simulink model "spot410_savedOnboard"  (R2024b)
settings: Solver=ode4  StartTime=0.0  StopTime=tsim  FixedStep=baseRate  RelTol=1e-6  AbsTol=1e-6
values from neighbouring files (symbols this model uses):
  baseRate = paramEst(phase,coord).k1    [SpotEstimator.m]
  Gamma1_el = 0.12    [initSpotDefaultParam.m]
  Gamma1_sh = 0.005    [initSpotDefaultParam.m]
  Gamma1_wr = 0.025    [initSpotDefaultParam.m]
  Gamma2_el = 5    [initSpotDefaultParam.m]
  Gamma2_sh = 5    [initSpotDefaultParam.m]
  Gamma2_wr = 5    [initSpotDefaultParam.m]
  Gamma3_el = 10    [initSpotDefaultParam.m]
  Gamma3_sh = 40    [initSpotDefaultParam.m]
  Gamma3_wr = 40    [initSpotDefaultParam.m]
  Gamma4_el = 0.039    [initSpotDefaultParam.m]
  Gamma4_sh = 0.015    [initSpotDefaultParam.m]
  Gamma4_wr = 0.029    [initSpotDefaultParam.m]
  Gamma5_el = 800    [initSpotDefaultParam.m]
  Gamma5_sh = 800    [initSpotDefaultParam.m]
  Gamma5_wr = 800    [initSpotDefaultParam.m]
  Gamma6_el = 0.000001    (= 1e-06)    [initSpotDefaultParam.m]
  Gamma6_sh = 0.005    [initSpotDefaultParam.m]
  Gamma6_wr = 0.02    [initSpotDefaultParam.m]
  Kd_elarm = 0.8    [initSpotDefaultParam.m]
  Kd_sharm = 1.0    (= 1)    [initSpotDefaultParam.m]
  Kd_wrarm = 0.6    [initSpotDefaultParam.m]
  Kp_elarm = 1.2    [initSpotDefaultParam.m]
  Kp_sharm = 1.5    [initSpotDefaultParam.m]
  Kp_wrarm = 1.0    (= 1)    [initSpotDefaultParam.m]
  PWMFreq = 5    [initSpotDefaultParam.m]
  Tz_lim_elarm = .1    (= 0.1)    [initSpotDefaultParam.m]
  Tz_lim_sharm = .1    (= 0.1)    [initSpotDefaultParam.m]
  Tz_lim_wrarm = .1    (= 0.1)    [initSpotDefaultParam.m]
undefined symbols (not defined in the file or in its folder): a1, a2, a3, b0, b1, b2, b3, dataRate, DiscIntNeverNeededParam, drop_states_ARM, drop_states_BLACK, drop_states_BLUE, drop_states_RED, F_black_X_nominal, F_black_Y_nominal, F_blue_X_nominal, F_blue_Y_nominal, F_red_X_nominal, F_red_Y_nominal, F_thrusters_BLACK, F_thrusters_BLUE, F_thrusters_RED, home_states_BLACK, home_states_BLUE, home_states_RED, IBLACK, IBLUE, IDIST, IEE, init_states_BLACK, init_states_BLUE, init_states_RED, IPROX, IRED, K_BLACK, K_BLUE, K_RED, Kd_tb, Kd_tblue, Kd_tr, Kd_xb, Kd_xblue, Kd_xr, Kd_yb, Kd_yblue, Kd_yr, Kp_tb, Kp_tblue, Kp_tr, Kp_xb, Kp_xblue, Kp_xr, Kp_yb, Kp_yblue, Kp_yr, mBLACK, mBLUE, mDIST, mEE, mPROX ... (+21)
libraries: simulink x30, nvidiaSharedBlocks x19, MainLibrary x5, dspinverses x3, nvidiaIMUSensorslib x1
(part 8 of 8)

== matlab function spot410_savedOnboard/Thruster Control Code/Change BLUE Behavior/Calculate Duty Cycle/MATLAB Function5 ==
  data: H_final output; u_desired input; duty_cycles output; x0 input; thruster_dist2CG_BLUE parameter; F_blue_X_nominal parameter; F_blue_Y_nominal parameter; max_iters parameter; tol parameter
function [H_final,duty_cycles] = optimize_duty_cycle_with_decay(u_desired, x0, thruster_dist2CG_BLUE, F_blue_X_nominal, F_blue_Y_nominal, max_iters, tol)
    % Optimizes thruster duty cycles with decay factor updates
    %
    % Inputs:
    %   u_desired - Desired force and torque vector [Fx; Fy; M] (3x1)
    %   x0 - Initial guess for duty cycles (vector, 8x1)
    %   max_iters - Maximum number of iterations for convergence
    %   tol - Convergence tolerance for duty cycles
    %   thruster_dist2CG_BLUE - Distances of thrusters from CG (vector, mm)
    %   F_red_X_nominal - Nominal X thruster force (scalar, N)
    %   F_red_Y_nominal - Nominal Y thruster force (scalar, N)
    %
    % Outputs:
    %   duty_cycles - Optimal duty cycles for each thruster (vector, 8x1)

    % Initialization
    num_thrusters = length(x0);
    duty_cycles = x0; % Start with the initial guess
    thrust_decay_factor = 1; % Initial decay factor
    prev_duty_cycles = duty_cycles + 2 * tol; % Ensure loop starts

    % Iterative optimization process
    for iter = 1:max_iters
        % Update H matrix based on the current decay factor
        H = MakeHWithDecay(thruster_dist2CG_BLUE, F_blue_X_nominal, thrust_decay_factor, F_blue_Y_nominal);
        
        % Define quadratic programming problem
        Q = 2 * (H' * H); % Quadratic term
        c = -2 * (H' * u_desired); % Linear term
        lb = zeros(num_thrusters, 1); % Lower bounds
        ub = ones(num_thrusters, 1); % Upper bounds
        options = optimoptions('quadprog', 'Display', 'off', 'Algorithm', 'active-set', 'MaxIterations', 5);
        
        % Solve for optimal duty cycles
        [duty_cycles, ~, ~] = quadprog(Q, c, [], [], [], [], lb, ub, duty_cycles, options);
        
        % Update decay factor based on the current duty cycles
        [thrust_decay_factor, ~] = check_thrust_decay(duty_cycles);
                
        % Check convergence criteria
        if norm(duty_cycles - prev_duty_cycles, Inf) < tol
            H_final = MakeHWithDecayRecalculateForce(thruster_dist2CG_BLUE, F_blue_X_nominal, thrust_decay_factor, F_blue_Y_nominal);
            return;
        end
            
        
        % Update for next iteration
        prev_duty_cycles = duty_cycles;
    end
    
    H_final = MakeHWithDecayRecalculateForce(thruster_dist2CG_BLUE, F_blue_X_nominal, thrust_decay_factor, F_blue_Y_nominal);
   

end

function H = MakeHWithDecay(thruster_dist2CG, F_X_nominal, thrust_decay_factor, F_Y_nominal)
    % Constructs the H matrix with thrust decay adjustments
    %
    % Inputs:
    %   thruster_dist2CG - Distances of thrusters from CG (vector, mm)
    %   F_X_nominal - Nominal X thruster force (scalar, N)
    %   thrust_decay_factor - Decay factor for thrust (scalar)
    %   F_Y_nominal - Nominal Y thruster force (scalar, N)
    %
    % Output:
    %   H - H matrix for optimization (3x8)

    % Adjust thruster distances (convert to meters)
    adjusted_thruster_dist2CG = thruster_dist2CG / 1000;

    % Define thruster contribution vectors
    Vec1 = [-1; -1;  0;  0;  1;  1;  0;  0]; % X-component
    Vec2 = [ 0;  0;  1;  1;  0;  0; -1; -1]; % Y-component
    Vec3 = adjusted_thruster_dist2CG;        % Moment arm (Z)

    % Combine vectors into the H matrix structure
    Mat1 = [Vec1, Vec2, Vec3]';
    
    % Adjust thruster forces with decay factor
    F_thrusters = [F_X_nominal; F_X_nominal; F_Y_nominal; F_Y_nominal; 
                   F_X_nominal; F_X_nominal; F_Y_nominal; F_Y_nominal] * thrust_decay_factor;

    % Scale forces for H matrix
    Mat2 = diag(F_thrusters / 2);

    % Compute final H matrix
    H = Mat1 * Mat2;
end

function H = MakeHWithDecayRecalculateForce(thruster_dist2CG, F_X_nominal, thrust_decay_factor, F_Y_nominal)
    % Constructs the H matrix with thrust decay adjustments
    %
    % Inputs:
    %   thruster_dist2CG - Distances of thrusters from CG (vector, mm)
    %   F_X_nominal - Nominal X thruster force (scalar, N)
    %   thrust_decay_factor - Decay factor for thrust (scalar)
    %   F_Y_nominal - Nominal Y thruster force (scalar, N)
    %
    % Output:
    %   H - H matrix for optimization (3x8)

    % Adjust thruster distances (convert to meters)
    adjusted_thruster_dist2CG = thruster_dist2CG / 1000;

    % Define thruster contribution vectors
    Vec1 = [-1; -1;  0;  0;  1;  1;  0;  0]; % X-component
    Vec2 = [ 0;  0;  1;  1;  0;  0; -1; -1]; % Y-component
    Vec3 = adjusted_thruster_dist2CG;        % Moment arm (Z)

    % Combine vectors into the H matrix structure
    Mat1 = [Vec1, Vec2, Vec3]';
    
    % Adjust thruster forces with decay factor
    F_thrusters = [F_X_nominal; F_X_nominal; F_Y_nominal; F_Y_nominal; 
                   F_X_nominal; F_X_nominal; F_Y_nominal; F_Y_nominal] * thrust_decay_factor;

    % Scale forces for H matrix
    Mat2 = diag(F_thrusters);

    % Compute final H matrix
    H = Mat1 * Mat2;
end

function [thrust_decay_factor, count] = check_thrust_decay(PWMs)
    % Updates the thrust decay factor based on current duty cycles
    %
    % Inputs:
    %   PWMs - Current duty cycle values (vector)
    %
    % Outputs:
    %   thrust_decay_factor - Updated decay factor (scalar)
    %   count - Number of active thrusters (scalar)

    % Normalize PWMs if necessary
    if max(PWMs) > 1
        PWMs = PWMs / max(PWMs);
    end

    % Count active thrusters
    count = sum(PWMs > 0);
    
    % Compute average duty cycle for active thrusters
    average_duty_cycle_per_thruster = sum(max(PWMs, 0)) / max(count, 1);

    % Update thrust decay factor based on average duty cycle
    if average_duty_cycle_per_thruster < 0.3 || count == 0
        thrust_decay_factor = 1;
    else
        thrust_decay_factor = max(0.6 - 2 * average_duty_cycle_per_thruster + 1, 0.5);
    end
end

== matlab function spot410_savedOnboard/Thruster Control Code/Change BLUE Behavior/Calculate Duty Cycle/Rotate Forces to Inertial/Create Rotation Matrix ==
  data: Rz input; C_Ib output
function C_Ib = RotateFrame(Rz)

C_bI = [  cos(Rz) sin(Rz)
         -sin(Rz) cos(Rz) ];

C_Ib = inv(C_bI);

end

== matlab function spot410_savedOnboard/Thruster Control Code/Change BLUE Behavior/Rotate Forces to Body/Create Rotation Matrix ==
  data: Rz input; C_bI output
function C_bI = RotateFrame(Rz)

C_bI = [  cos(Rz) sin(Rz)
         -sin(Rz) cos(Rz) ];

end

== matlab function spot410_savedOnboard/Thruster Control Code/Change RED Behavior/Calculate Duty Cycle/Generate Initial Guess/MATLAB Function ==
  data: H output; thruster_dist2CG_RED parameter; F_thrusters_RED parameter
function H = MakeH(thruster_dist2CG_RED,F_thrusters_RED)

    Vec1 = [ -1
             -1
              0 
              0
              1
              1
              0
              0 ];
          
    Vec2 = [  0
              0
              1
              1
              0
              0
             -1
             -1 ];
         
    Vec3 = thruster_dist2CG_RED./1000;
    
    Mat1 = [Vec1, Vec2, Vec3]';
    
    Mat2 = diag((F_thrusters_RED./2));
    
    H    = Mat1*Mat2;

end

== matlab function spot410_savedOnboard/Thruster Control Code/Change RED Behavior/Calculate Duty Cycle/MATLAB Function5 ==
  data: H_final output; u_desired input; duty_cycles output; x0 input; thruster_dist2CG_RED parameter; F_red_X_nominal parameter; F_red_Y_nominal parameter; max_iters parameter; tol parameter
function [H_final,duty_cycles] = optimize_duty_cycle_with_decay(u_desired, x0, thruster_dist2CG_RED, F_red_X_nominal, F_red_Y_nominal, max_iters, tol)
    % Optimizes thruster duty cycles with decay factor updates
    %
    % Inputs:
    %   u_desired - Desired force and torque vector [Fx; Fy; M] (3x1)
    %   x0 - Initial guess for duty cycles (vector, 8x1)
    %   max_iters - Maximum number of iterations for convergence
    %   tol - Convergence tolerance for duty cycles
    %   thruster_dist2CG_RED - Distances of thrusters from CG (vector, mm)
    %   F_red_X_nominal - Nominal X thruster force (scalar, N)
    %   F_red_Y_nominal - Nominal Y thruster force (scalar, N)
    %
    % Outputs:
    %   duty_cycles - Optimal duty cycles for each thruster (vector, 8x1)

    % Initialization
    num_thrusters = length(x0);
    duty_cycles = x0; % Start with the initial guess
    thrust_decay_factor = 1; % Initial decay factor
    prev_duty_cycles = duty_cycles + 2 * tol; % Ensure loop starts

    % Iterative optimization process
    for iter = 1:max_iters
        % Update H matrix based on the current decay factor
        H = MakeHWithDecay(thruster_dist2CG_RED, F_red_X_nominal, thrust_decay_factor, F_red_Y_nominal);
        
        % Define quadratic programming problem
        Q = 2 * (H' * H); % Quadratic term
        c = -2 * (H' * u_desired); % Linear term
        lb = zeros(num_thrusters, 1); % Lower bounds
        ub = ones(num_thrusters, 1); % Upper bounds
        options = optimoptions('quadprog', 'Display', 'off', 'Algorithm', 'active-set', 'MaxIterations', 5);
        
        % Solve for optimal duty cycles
        [duty_cycles, ~, ~] = quadprog(Q, c, [], [], [], [], lb, ub, duty_cycles, options);
        
        % Update decay factor based on the current duty cycles
        [thrust_decay_factor, ~] = check_thrust_decay(duty_cycles);
                
        % Check convergence criteria
        if norm(duty_cycles - prev_duty_cycles, Inf) < tol
            H_final = MakeHWithDecayRecalculateForce(thruster_dist2CG_RED, F_red_X_nominal, thrust_decay_factor, F_red_Y_nominal);
            return;
        end
            
        
        % Update for next iteration
        prev_duty_cycles = duty_cycles;
    end
    
    H_final = MakeHWithDecayRecalculateForce(thruster_dist2CG_RED, F_red_X_nominal, thrust_decay_factor, F_red_Y_nominal);
   

end

function H = MakeHWithDecay(thruster_dist2CG, F_X_nominal, thrust_decay_factor, F_Y_nominal)
    % Constructs the H matrix with thrust decay adjustments
    %
    % Inputs:
    %   thruster_dist2CG - Distances of thrusters from CG (vector, mm)
    %   F_X_nominal - Nominal X thruster force (scalar, N)
    %   thrust_decay_factor - Decay factor for thrust (scalar)
    %   F_Y_nominal - Nominal Y thruster force (scalar, N)
    %
    % Output:
    %   H - H matrix for optimization (3x8)

    % Adjust thruster distances (convert to meters)
    adjusted_thruster_dist2CG = thruster_dist2CG / 1000;

    % Define thruster contribution vectors
    Vec1 = [-1; -1;  0;  0;  1;  1;  0;  0]; % X-component
    Vec2 = [ 0;  0;  1;  1;  0;  0; -1; -1]; % Y-component
    Vec3 = adjusted_thruster_dist2CG;        % Moment arm (Z)

    % Combine vectors into the H matrix structure
    Mat1 = [Vec1, Vec2, Vec3]';
    
    % Adjust thruster forces with decay factor
    F_thrusters = [F_X_nominal; F_X_nominal; F_Y_nominal; F_Y_nominal; 
                   F_X_nominal; F_X_nominal; F_Y_nominal; F_Y_nominal] * thrust_decay_factor;

    % Scale forces for H matrix
    Mat2 = diag(F_thrusters / 2);

    % Compute final H matrix
    H = Mat1 * Mat2;
end

function H = MakeHWithDecayRecalculateForce(thruster_dist2CG, F_X_nominal, thrust_decay_factor, F_Y_nominal)
    % Constructs the H matrix with thrust decay adjustments
    %
    % Inputs:
    %   thruster_dist2CG - Distances of thrusters from CG (vector, mm)
    %   F_X_nominal - Nominal X thruster force (scalar, N)
    %   thrust_decay_factor - Decay factor for thrust (scalar)
    %   F_Y_nominal - Nominal Y thruster force (scalar, N)
    %
    % Output:
    %   H - H matrix for optimization (3x8)

    % Adjust thruster distances (convert to meters)
    adjusted_thruster_dist2CG = thruster_dist2CG / 1000;

    % Define thruster contribution vectors
    Vec1 = [-1; -1;  0;  0;  1;  1;  0;  0]; % X-component
    Vec2 = [ 0;  0;  1;  1;  0;  0; -1; -1]; % Y-component
    Vec3 = adjusted_thruster_dist2CG;        % Moment arm (Z)

    % Combine vectors into the H matrix structure
    Mat1 = [Vec1, Vec2, Vec3]';
    
    % Adjust thruster forces with decay factor
    F_thrusters = [F_X_nominal; F_X_nominal; F_Y_nominal; F_Y_nominal; 
                   F_X_nominal; F_X_nominal; F_Y_nominal; F_Y_nominal] * thrust_decay_factor;

    % Scale forces for H matrix
    Mat2 = diag(F_thrusters);

    % Compute final H matrix
    H = Mat1 * Mat2;
end

function [thrust_decay_factor, count] = check_thrust_decay(PWMs)
    % Updates the thrust decay factor based on current duty cycles
    %
    % Inputs:
    %   PWMs - Current duty cycle values (vector)
    %
    % Outputs:
    %   thrust_decay_factor - Updated decay factor (scalar)
    %   count - Number of active thrusters (scalar)

    % Normalize PWMs if necessary
    if max(PWMs) > 1
        PWMs = PWMs / max(PWMs);
    end

    % Count active thrusters
    count = sum(PWMs > 0);
    
    % Compute average duty cycle for active thrusters
    average_duty_cycle_per_thruster = sum(max(PWMs, 0)) / max(count, 1);

    % Update thrust decay factor based on average duty cycle
    if average_duty_cycle_per_thruster < 0.3 || count == 0
        thrust_decay_factor = 1;
    else
        thrust_decay_factor = max(0.6 - 2 * average_duty_cycle_per_thruster + 1, 0.5);
    end
end

== matlab function spot410_savedOnboard/Thruster Control Code/Change RED Behavior/Calculate Duty Cycle/Rotate Forces to Inertial/Create Rotation Matrix ==
  data: Rz input; C_Ib output
function C_Ib = RotateFrame(Rz)

C_bI = [  cos(Rz) sin(Rz)
         -sin(Rz) cos(Rz) ];

C_Ib = inv(C_bI);

end

== matlab function spot410_savedOnboard/Thruster Control Code/Change RED Behavior/Rotate Forces to Body/Create Rotation Matrix ==
  data: Rz input; C_bI output
function C_bI = RotateFrame(Rz)

C_bI = [  cos(Rz) sin(Rz)
         -sin(Rz) cos(Rz) ];

end

== matlab function spot410_savedOnboard/SpotGnc/SpotEstimator ==
  data: phase input; proc input; cmd input; est output; est_vel output; paramEst parameter; est_bias output; debug output
function [est,est_vel,est_bias,debug] = SpotEstimator(phase, proc, cmd, paramEst)

    [est,est_vel,est_bias,debug] = SpotEstimator(phase, proc, cmd, paramEst);

end

== matlab function spot410_savedOnboard/Thruster Control Code/Change BLACK Behavior/Calculate Duty Cycle/MATLAB Function1 ==
  data: ThrustPer_Final output; ThrustPer input; PWMFreq parameter
function ThrustPer_Final  = ThrusterSat(ThrustPer, PWMFreq)

    ValveTime       = 0.007;
    TControl        = 1/PWMFreq;

    ThrustPer_Final = zeros(8,1);
    
    if max(ThrustPer) > 1
        ThrustPer_Sat = ThrustPer/max(ThrustPer);
    else
        ThrustPer_Sat = ThrustPer;
    end
    
    for i = 1:8
        if ThrustPer_Sat(i) > ValveTime/TControl 
            ThrustPer_Final(i) = ThrustPer_Sat(i);
        else
            ThrustPer_Final(i) = 0;
        end
    end


end

== matlab function spot410_savedOnboard/Thruster Control Code/Change RED Behavior/Calculate Duty Cycle/MATLAB Function8 ==
  data: ThrustPer_Final output; ThrustPer input; PWMFreq parameter
function ThrustPer_Final  = ThrusterSat(ThrustPer, PWMFreq)

    ValveTime       = 0.007;
    TControl        = 1/PWMFreq;

    ThrustPer_Final = zeros(8,1);
    
    if max(ThrustPer) > 1
        ThrustPer_Sat = ThrustPer/max(ThrustPer);
    else
        ThrustPer_Sat = ThrustPer;
    end
    
    for i = 1:8
        if ThrustPer_Sat(i) > ValveTime/TControl 
            ThrustPer_Final(i) = ThrustPer_Sat(i);
        else
            ThrustPer_Final(i) = 0;
        end
    end


end

== matlab function spot410_savedOnboard/SpotGnc/SpotRefGen ==
  data: phase input; t input; proc input; ref output; paramRefGen parameter; ref_vel output
function [ref,ref_vel] = SpotRefGen(phase, t, proc, paramRefGen)

    [ref,ref_vel] = SpotRefGen(phase, t, proc, paramRefGen);

end

== matlab function spot410_savedOnboard/Simulate Plant Dynamics/RED and ARM Dynamics/RED + ARM/Dynamics Model ==
  data: q_dot output; x input; InertiaS input; CoriolisS input; u input; Gamma1_sh parameter; Gamma2_sh parameter; Gamma3_sh parameter; Gamma5_sh parameter; Gamma4_sh parameter; Gamma6_sh parameter; Gamma1_el parameter; Gamma2_el parameter; Gamma3_el parameter; Gamma5_el parameter; Gamma4_el parameter; Gamma6_el parameter; Gamma1_wr parameter; Gamma2_wr parameter; Gamma3_wr parameter; Gamma5_wr parameter; Gamma4_wr parameter; Gamma6_wr parameter; q_ddot output
function [q_dot, q_ddot]  = DynamicsModel(x, InertiaS, CoriolisS, u,...
    Gamma1_sh, Gamma2_sh, Gamma3_sh, Gamma5_sh, Gamma4_sh, Gamma6_sh,...
    Gamma1_el, Gamma2_el, Gamma3_el, Gamma5_el, Gamma4_el, Gamma6_el,...
    Gamma1_wr, Gamma2_wr, Gamma3_wr, Gamma5_wr, Gamma4_wr, Gamma6_wr)


    fqdot1 = Gamma1_sh*(tanh(Gamma2_sh*x(10)) - tanh(Gamma3_sh*x(10))) + Gamma4_sh*tanh(Gamma5_sh*x(10)) + Gamma6_sh*x(10);

    fqdot2 = Gamma1_el*(tanh(Gamma2_el*x(11)) - tanh(Gamma3_el*x(11))) + Gamma4_el*tanh(Gamma5_el*x(11)) + Gamma6_el*x(11);

    fqdot3 = Gamma1_wr*(tanh(Gamma2_wr*x(12)) - tanh(Gamma3_wr*x(12))) + Gamma4_wr*tanh(Gamma5_wr*x(12)) + Gamma6_wr*x(12);
    
    q_dot  = x(7:12);
    q_ddot = pinv(InertiaS)*(u - CoriolisS*x(7:12) - [0;0;0;fqdot1;fqdot2;fqdot3]);
    
end

== matlab function spot410_savedOnboard/SpotGnc/MATLAB Function ==
  data: phase input; puckState output; armState output; paramFlag parameter
function [puckState,armState] = SpotFlag(phase, paramFlag)

    [puckState,armState] = SpotFlag(phase, paramFlag);

end

== matlab function spot410_savedOnboard/Thruster Control Code/Change BLUE Behavior/Calculate Duty Cycle/MATLAB Function1 ==
  data: ThrustPer_Final output; ThrustPer input; PWMFreq parameter
function ThrustPer_Final  = ThrusterSat(ThrustPer, PWMFreq)

    ValveTime       = 0.007;
    TControl        = 1/PWMFreq;

    ThrustPer_Final = zeros(8,1);
    
    if max(ThrustPer) > 1
        ThrustPer_Sat = ThrustPer/max(ThrustPer);
    else
        ThrustPer_Sat = ThrustPer;
    end
    
    for i = 1:8
        if ThrustPer_Sat(i) > ValveTime/TControl 
            ThrustPer_Final(i) = ThrustPer_Sat(i);
        else
            ThrustPer_Final(i) = 0;
        end
    end


end

== matlab function spot410_savedOnboard/SpotGnc/MATLAB Function1 ==
  data: t input; phase output; paramPhaseMgmt parameter
function phase  = SpotPhaseMgmt(t, paramPhaseMgmt)

    [phase] = SpotPhaseMgmt(t, paramPhaseMgmt);

end

== matlab function spot410_savedOnboard/PhaseSpace Camera Code/Use Hardware to Obtain States/Receive and Process Phasespace Data/Check for Sychronization/MATLAB Function ==
  data: StartClock output; RedReceiving input; BlackReceiving input; BlueReceiving input; platformSelection parameter
function StartClock = CheckForSync(RedReceiving, BlackReceiving, BlueReceiving, platformSelection)
        
    StartClock = 0;
    
    if (platformSelection == 1)
        
        if RedReceiving == 1

            StartClock = 1;

        else

            StartClock = 0;

        end
        
    elseif (platformSelection == 2)
        
        if BlackReceiving == 1

            StartClock = 1;

        else

            StartClock = 0;

        end  
        
    elseif (platformSelection == 3)
        
        if RedReceiving == 1 && BlackReceiving == 1

            StartClock = 1;

        else

            StartClock = 0;

        end    
        
    elseif (platformSelection == 4)
        
        if RedReceiving == 1 && BlackReceiving == 1

            StartClock = 1;

        else

            StartClock = 0;

        end
        
    elseif (platformSelection == 5)
        
        if RedReceiving == 1

            StartClock = 1;

        else

            StartClock = 0;

        end
        
    elseif (platformSelection == 6)
        
        if BlueReceiving == 1

            StartClock = 1;

        else

            StartClock = 0;

        end
        
    elseif (platformSelection == 7)
        
        if RedReceiving == 1 && BlueReceiving == 1

            StartClock = 1;

        else

            StartClock = 0;

        end
        
    elseif (platformSelection == 8)
        
        if RedReceiving == 1 && BlackReceiving == 1 && BlueReceiving == 1

            StartClock = 1;

        else

            StartClock = 0;

        end
        
    elseif (platformSelection == 9)
        
        if BlackReceiving == 1 && BlueReceiving == 1

            StartClock = 1;

        else

            StartClock = 0;

        end
                           
    elseif (platformSelection == 10)
        
        if RedReceiving == 1 && BlueReceiving == 1

            StartClock = 1;

        else

            StartClock = 0;

        end
        
    elseif (platformSelection == 11)
        
        if RedReceiving == 1 && BlackReceiving == 1 && BlueReceiving == 1

            StartClock = 1;

        else

            StartClock = 0;

        end
        
    end



end

== matlab function spot410_savedOnboard/3 - Control/Default LQR Control (RED)/Calculate Error/MATLAB Function ==
  data: Rz_path input; Rz_error output; Rz_measured input
function Rz_error = SmoothAngularDifference(Rz_path, Rz_measured)

    Rz_error = mod(Rz_measured-Rz_path+pi, 2*pi)-pi;


end

== matlab function spot410_savedOnboard/3 - Control/Default LQR Control (BLACK)/Calculate Error/MATLAB Function ==
  data: Rz_path input; Rz_error output; Rz_measured input
function Rz_error = SmoothAngularDifference(Rz_path, Rz_measured)

    Rz_error = mod(Rz_measured-Rz_path+pi, 2*pi)-pi;


end

== matlab function spot410_savedOnboard/3 - Control/Default PD Control (RED)/Calculate Error/MATLAB Function ==
  data: Rz_path input; Rz_error output; Rz_measured input
function Rz_error = SmoothAngularDifference(Rz_path, Rz_measured)

    Rz_error = mod(Rz_measured-Rz_path+pi, 2*pi)-pi;


end
